simulink model "RC"  (R2017a)
settings: Solver=FixedStepAuto  StartTime=0.0  StopTime=86400  FixedStep=1  MaxStep=1e-4  RelTol=1e-3
settings Model: Creator=Pepe  LastModifiedBy=Pepe
settings DebuggingCC: UnconnectedInputMsg=none  UnconnectedOutputMsg=none  UnconnectedLineMsg=none

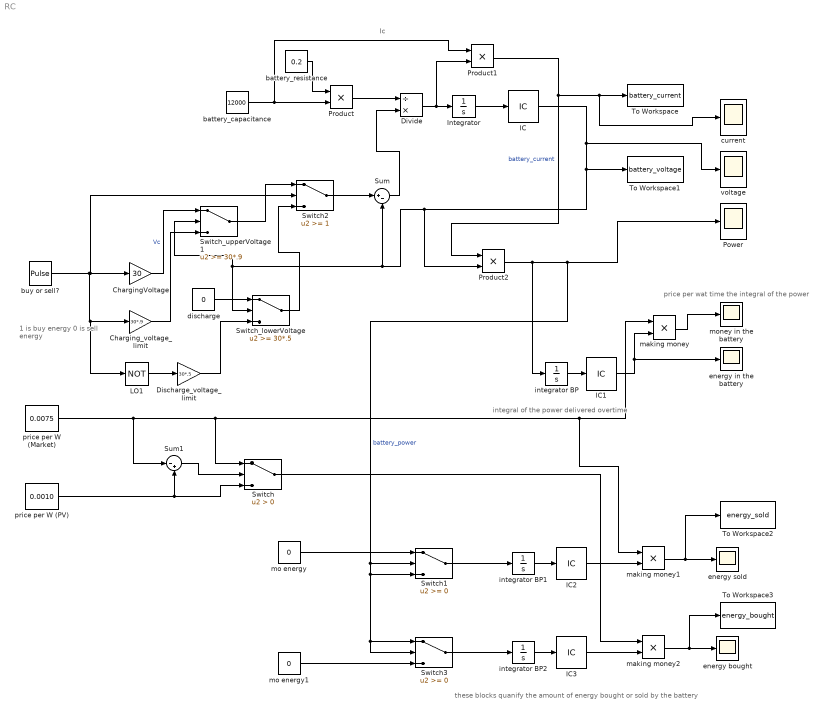
== system RC ==
  note: 1 is buy energy
      | 0 is sell energy
  note: these blocks quanify the amount of energy bought or sold by the battery
  note: integral of the power delivered overtime
  note: price per wat time the integral of the power
  note: Ic
  "ChargingVoltage " : Gain  Gain=30
  "Charging_voltage_limit " : Gain  Gain=30*.9
  Discharge_voltage_limit : Gain  Gain=30*.5
  Divide : Product  Inputs=/*
  IC{,1..3} (4 alike) : InitialCondition  Value=0
  Integrator : Integrator  InitialCondition=30*.2
  LO1 : Logic  Operator=NOT  AllPortsSameDT=off  OutDataTypeStr=boolean
  Power : Scope
  Product : Product
  Product1 : Product
  Product2 : Product
  Sum : Sum  Inputs=|+-
  Sum1 : Sum  Inputs=|-+
  Switch : Switch  Criteria=u2 > Threshold
  Switch1 : Switch
      settings: LockScale=on
  Switch2 : Switch  Threshold=1
      settings: LockScale=on
  Switch3 : Switch
      settings: LockScale=on
  Switch_lowerVoltage : Switch  Threshold=30*.5
  Switch_upperVoltage1 : Switch  Threshold=30*.9
  To Workspace : ToWorkspace  VariableName=battery_current  SaveFormat=Timeseries  SampleTime=-1
  To Workspace1 : ToWorkspace  VariableName=battery_voltage  SaveFormat=Timeseries  SampleTime=-1
  To Workspace2 : ToWorkspace  VariableName=energy_sold  SaveFormat=Timeseries  SampleTime=-1
  To Workspace3 : ToWorkspace  VariableName=energy_bought  SaveFormat=Timeseries  SampleTime=-1
  battery_capacitance : Constant  Value=12000
  battery_resistance : Constant  Value=0.2
  buy or sell? : DiscretePulseGenerator  PulseType=Time based  Period=2400*5  PulseWidth=50
  "current " : Scope
  discharge : Constant  Value=0
  energy bought : Scope
  energy in the battery : Scope
  energy sold : Scope
  integrator BP : Integrator  InitialCondition=30*.2
  integrator BP1 : Integrator  InitialCondition=30*.2
  integrator BP2 : Integrator  InitialCondition=30*.2
  making money : Product
  making money1 : Product
  making money2 : Product
  mo energy : Constant  Value=0
  mo energy1 : Constant  Value=0
  money in the battery : Scope
  price per W (Market) : Constant  Value=0.0075
  price per W (PV) : Constant  Value=0.0010
  voltage : Scope
  wires:
  battery_resistance/1 -> Product/1
  Product/1 -> Divide/1
  Sum/1 -> Divide/2
  Divide/1 -> Product1/2, Integrator/1
  Integrator/1 -> IC/1
  IC/1 -> voltage/1, Product2/2, Sum/2, Switch_upperVoltage1/2, Switch_lowerVoltage/2, To Workspace1/1
  Product2/1 -> Switch3/1, Switch3/2, Switch1/3, Switch1/2, Power/1, integrator BP/1  "battery_power"
  battery_capacitance/1 -> Product/2, Product1/1
  Product1/1 -> Product2/1, "current "/1, To Workspace/1  "battery_current"
  buy or sell?/1 -> LO1/1, "Charging_voltage_limit "/1, Switch2/2, "ChargingVoltage "/1
  "Charging_voltage_limit "/1 -> Switch_upperVoltage1/3
  LO1/1 -> Discharge_voltage_limit/1
  Switch_lowerVoltage/1 -> Switch2/3
  Discharge_voltage_limit/1 -> Switch_lowerVoltage/3
  "ChargingVoltage "/1 -> Switch_upperVoltage1/1  "Vc"
  Switch2/1 -> Sum/1
  Switch_upperVoltage1/1 -> Switch2/1
  discharge/1 -> Switch_lowerVoltage/1
  integrator BP/1 -> IC1/1
  IC1/1 -> making money/2, energy in the battery/1
  price per W (Market)/1 -> Sum1/1, Switch/1, making money1/1, making money/1
  making money/1 -> money in the battery/1
  Switch1/1 -> integrator BP1/1
  integrator BP1/1 -> IC2/1
  making money1/1 -> To Workspace2/1, energy sold/1
  IC2/1 -> making money1/2
  mo energy/1 -> Switch1/1
  integrator BP2/1 -> IC3/1
  making money2/1 -> To Workspace3/1, energy bought/1
  Switch3/1 -> integrator BP2/1
  IC3/1 -> making money2/2
  mo energy1/1 -> Switch3/3
  price per W (PV)/1 -> Sum1/2, Switch/3
  Sum1/1 -> Switch/2
  Switch/1 -> making money2/1
